simulink model "HIL_PID"  (R2025b)
settings: Solver=FixedStepDiscrete  StartTime=0.0  StopTime=10.0  FixedStep=0.01  RelTol=1e-3
model workspace (MAT data in the model file):
  K = 126
  tau = 0.1
settings Model: Creator=joshc  LastModifiedBy=joshc

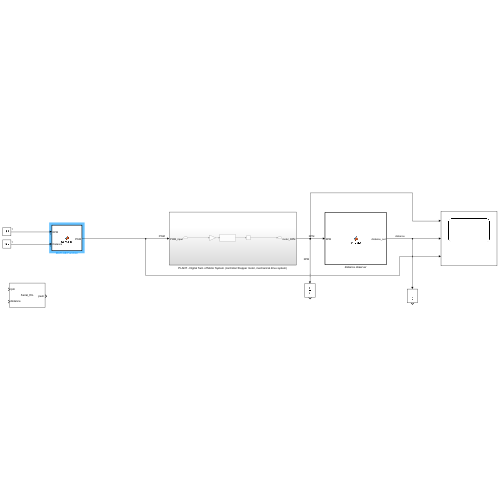
[thumbnail: Simulink's stored preview of the top-level diagram]
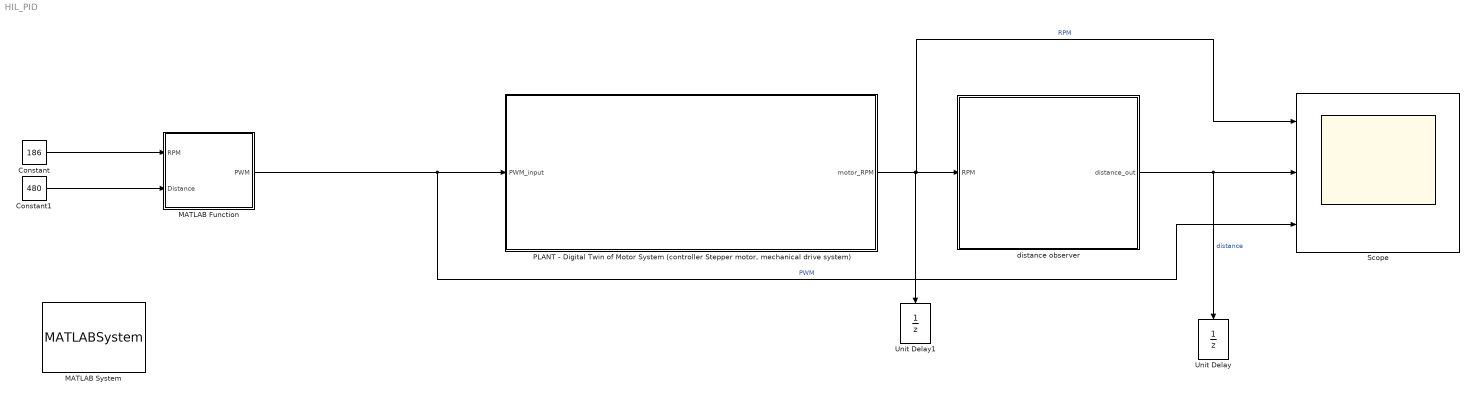
== system HIL_PID ==
  Constant : Constant  Value=186  SampleTime=0.1
  Constant1 : Constant  Value=480  SampleTime=0.01
  MATLAB Function : MATLAB Function  TreatAsAtomicUnit=on
  MATLAB System : MATLABSystem  System=Serial_HIL  Port=COM9  BaudRate=2000000  SimulateUsing=Interpreted execution
      mask Type: Serial_HIL
  "PLANT - Digital Twin of Motor System (controller Stepper motor, mechanical drive system)" : Subsystem
  Scope : Scope  NumInputPorts=3
      settings: ActiveDisplayYMinimum=-51.4383436154113  ActiveDisplayYMaximum=900.85315452025054
  Unit Delay : UnitDelay  SampleTime=0.01  HasFrameUpgradeWarning=on
  Unit Delay1 : UnitDelay  SampleTime=0.01  HasFrameUpgradeWarning=on
  distance observer : MATLAB Function  TreatAsAtomicUnit=on
  wires:
  MATLAB Function/1(PWM) -> Scope/3, "PLANT - Digital Twin of Motor System (controller Stepper motor, mechanical drive system)"/1(PWM_input)  "PWM"
  "PLANT - Digital Twin of Motor System (controller Stepper motor, mechanical drive system)"/1(motor_RPM) -> Scope/1, distance observer/1(RPM), Unit Delay1/1  "RPM"
  distance observer/1(distance_out) -> Unit Delay/1, Scope/2  "distance"
  Constant/1 -> MATLAB Function/1(RPM)
  Constant1/1 -> MATLAB Function/2(Distance)

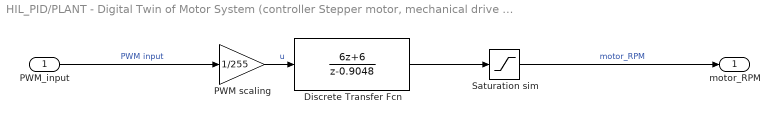
== system HIL_PID/PLANT - Digital Twin of Motor System (controller Stepper motor, mechanical drive system) ==
  PWM_input : Inport
  Discrete Transfer Fcn : DiscreteTransferFcn  Numerator=[6,6]  Denominator=[1, -0.9048]
  PWM scaling : Gain  Gain=1/255
  Saturation sim : Saturate  UpperLimit=186  LowerLimit=0
  motor_RPM : Outport
  wires:
  PWM_input/1 -> PWM scaling/1  "PWM input"
  PWM scaling/1 -> Discrete Transfer Fcn/1  "u"
  Discrete Transfer Fcn/1 -> Saturation sim/1
  Saturation sim/1 -> motor_RPM/1  "motor_RPM"

== matlab function HIL_PID/MATLAB Function ==
  data: RPM input; PWM output; Distance input
function PWM = SerialHIL(RPM, Distance)
% SerialHIL communicates with the ESP32 to send RPM & Distance and receive PWM
% Inputs:
%   RPM      - measured or reference RPM
%   Distance - measured or reference distance
% Output:
%   PWM      - PWM returned from ESP32

    % Persistent serial object
    persistent s
    if isempty(s)
        s = serialport("COM9", 2000000); % Set your COM port & baud rate
        configureTerminator(s,"LF");
        flush(s);
    end

    % Default output
    PWM = 0;

    try
        % Send RPM and Distance to ESP32
        msg = sprintf('%.2f,%.2f\n', RPM, Distance);
        write(s, uint8(msg), 'uint8'); % Send as bytes

        % Read PWM from ESP32 if available
        if s.NumBytesAvailable > 0
            line = readline(s);      % Read until '\n'
            PWM = str2double(line);  % Convert to numeric
        end
    catch ME
        % Optional: display warning instead of crashing Simulink
        warning('Serial communication error: %s', E.message);
    end
end

== matlab function HIL_PID/distance observer ==
  settings: updateMethod=DISCRETE
  data: RPM input; distance_out output
function distance_out = rpm2dist(RPM)
    diameter = 49.7;
    Ts = 0.01;
    circumference = pi*diameter;

    persistent x last_distance
    if isempty(x)
        x = 0;
    end
    if isempty(last_distance)
        last_distance = 0;
    end

    speed = (RPM/60)*circumference;
    x = x + speed*Ts;

    distance_out = last_distance;   % output previous step
    last_distance = x;              % store for next step
end
